simulink model "sf_slswitch_nk"  (R2020a)
settings: Solver=FixedStepAuto  StartTime=0.0  StopTime=options.T_train  FixedStep=options.dt  MaxStep=.2  RelTol=1e-3
model workspace (MAT data in the model file):
  PID_TRESH = 0.3
values from neighbouring files (symbols this model uses):
  options = trainingOptions('sgdm',      'MiniBatchSize',miniBatchSize,      'MaxEpochs',30,      'InitialLearnRate',1e-3,      'LearnRateSchedule','piecewise',      'LearnRateDropFactor',0.1,      'LearnRateDropPeriod',20,      'Shuffle','every-epoch',      'ValidationData',{XValidation,YValidation},      'ValidationFrequency',validationFrequency,      'Plots','training-progress',      'Verbose',false)    [training_lstm.m]
undefined symbols (not defined in the file or in its folder): DiscIntNeverNeededParam
libraries: neural x72, simulink x3
(part 2 of 3)

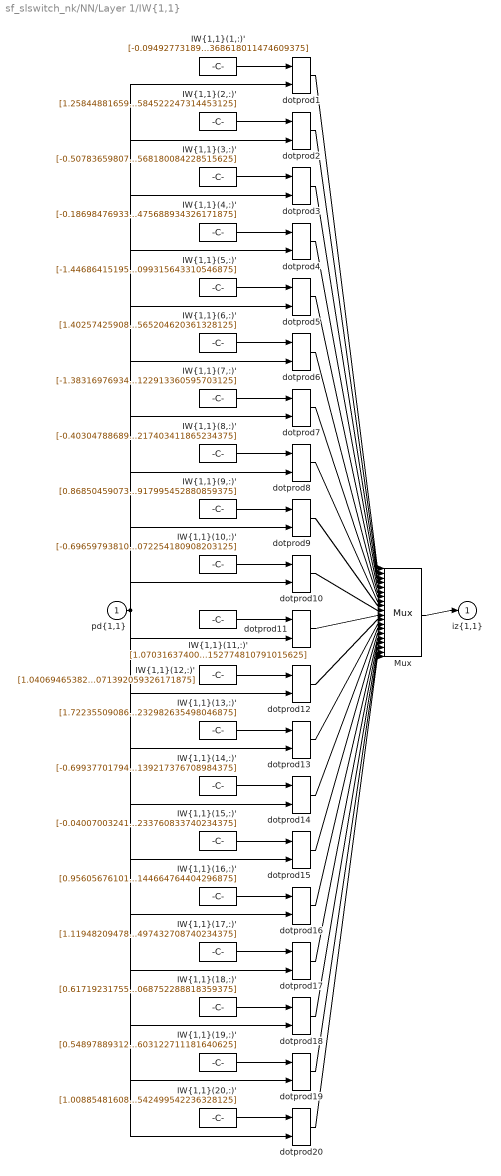
== system sf_slswitch_nk/NN/Layer 1/IW{1,1} ==
  "pd{1,1}" : Inport  PortDimensions=6
      mask Display: e = 0.06;c1 = [120 230 180]/255;c2 = ([120 230 180]+0)/(256+128);c3 = ([120 230 180]+128)/(256+128);patch([0 1 1 0],[0 0 1 1],c1);patch([0 1 1 1-e 1-e 0+e],[0 0 1 1-e 0+e 0+e],c2);patch([0 0 1 1-e 0+e 0+e],[0 1 1 1-e 1-e 0+e],c3);plot([0 1 1 0 0],[0 0 1 1 0]);
  "IW{1,1}(1,:)'" : Constant  Value=[-0.094927731895724232202837811200879514217376708984375;-1.078124816183085865617385934456251561641693115234375;-0.294993423128365128693673113957629539072513580322265625;1.256774030726915736266846579383127391338348388671875;-1.067658796670704735021217857138253748416900634765625;-0.36738733480733321012934311511344276368618011474609375]
      mask Display: e = 0.06;c1 = [120 150 230]/255;c2 = ([120 150 230]+0)/383;c3 = ([120 150 230]+128)/383;patch([0 1 1 0],[0 0 1 1],c1);patch([0 1 1 1-e 1-e 0+e],[0 0 1 1-e 0+e 0+e],c2);patch([0 0 1 1-e 0+e 0+e],[0 1 1 1-e 1-e 0+e],c3);plot([0 1 1 0 0],[0 0 1 1 0]);disp('Weights');
  "IW{1,1}(10,:)'" : Constant  Value=[-0.6965979381092519684415265146526508033275604248046875;-0.93137227491803764589661795980646274983882904052734375;-1.6314384415528950800222673933603800833225250244140625;0.32289582670247385376427473602234385907649993896484375;1.291547019617809155533905141055583953857421875;1.45726842545820733931805079919286072254180908203125]
      mask Display: e = 0.06;c1 = [120 150 230]/255;c2 = ([120 150 230]+0)/383;c3 = ([120 150 230]+128)/383;patch([0 1 1 0],[0 0 1 1],c1);patch([0 1 1 1-e 1-e 0+e],[0 0 1 1-e 0+e 0+e],c2);patch([0 0 1 1-e 0+e 0+e],[0 1 1 1-e 1-e 0+e],c3);plot([0 1 1 0 0],[0 0 1 1 0]);disp('Weights');
  "IW{1,1}(11,:)'" : Constant  Value=[1.07031637400404111559737430070526897907257080078125;-0.9847080253491229395734762874781154096126556396484375;-0.61960709489012832928978014024323783814907073974609375;1.0400372152841772521725260958191938698291778564453125;0.89700998933492004372425299152382649481296539306640625;-1.3575066104025721447357000215561129152774810791015625]
      mask Display: e = 0.06;c1 = [120 150 230]/255;c2 = ([120 150 230]+0)/383;c3 = ([120 150 230]+128)/383;patch([0 1 1 0],[0 0 1 1],c1);patch([0 1 1 1-e 1-e 0+e],[0 0 1 1-e 0+e 0+e],c2);patch([0 0 1 1-e 0+e 0+e],[0 1 1 1-e 1-e 0+e],c3);plot([0 1 1 0 0],[0 0 1 1 0]);disp('Weights');
  "IW{1,1}(12,:)'" : Constant  Value=[1.0406946538218460052149794137221761047840118408203125;-0.693594025462512586699403982493095099925994873046875;0.468858240358544176018540383665822446346282958984375;0.68547826794217259216424054102390073239803314208984375;-0.7853865691300843110411733505316078662872314453125;-1.8329776342435948333076112248818390071392059326171875]
      mask Display: e = 0.06;c1 = [120 150 230]/255;c2 = ([120 150 230]+0)/383;c3 = ([120 150 230]+128)/383;patch([0 1 1 0],[0 0 1 1],c1);patch([0 1 1 1-e 1-e 0+e],[0 0 1 1-e 0+e 0+e],c2);patch([0 0 1 1-e 0+e 0+e],[0 1 1 1-e 1-e 0+e],c3);plot([0 1 1 0 0],[0 0 1 1 0]);disp('Weights');
  "IW{1,1}(13,:)'" : Constant  Value=[1.72235509086079918716905012843199074268341064453125;-0.83361662074459186300146029680036008358001708984375;0.466763693573051419161146213809843175113201141357421875;-1.5345239974877646904616312895086593925952911376953125;-0.404560405975131487377183248099754564464092254638671875;0.421133717269054130838412675075232982635498046875]
      mask Display: e = 0.06;c1 = [120 150 230]/255;c2 = ([120 150 230]+0)/383;c3 = ([120 150 230]+128)/383;patch([0 1 1 0],[0 0 1 1],c1);patch([0 1 1 1-e 1-e 0+e],[0 0 1 1-e 0+e 0+e],c2);patch([0 0 1 1-e 0+e 0+e],[0 1 1 1-e 1-e 0+e],c3);plot([0 1 1 0 0],[0 0 1 1 0]);disp('Weights');
  "IW{1,1}(14,:)'" : Constant  Value=[-0.6993770179442133638758605229668319225311279296875;-0.67988096027652022979026469329255633056163787841796875;1.72051357171069785323425094247795641422271728515625;0.8663489352893309902725604842999018728733062744140625;0.088446533921556935720076353391050361096858978271484375;-1.4915026481155793103283713207929395139217376708984375]
      mask Display: e = 0.06;c1 = [120 150 230]/255;c2 = ([120 150 230]+0)/383;c3 = ([120 150 230]+128)/383;patch([0 1 1 0],[0 0 1 1],c1);patch([0 1 1 1-e 1-e 0+e],[0 0 1 1-e 0+e 0+e],c2);patch([0 0 1 1-e 0+e 0+e],[0 1 1 1-e 1-e 0+e],c3);plot([0 1 1 0 0],[0 0 1 1 0]);disp('Weights');
  "IW{1,1}(15,:)'" : Constant  Value=[-0.04007003241597495435399878260795958340167999267578125;-0.64990767603311094813278714354964904487133026123046875;1.57234891421088374130476950085721909999847412109375;0.9274205308829746030596652417443692684173583984375;-1.00715212796622921587186283431947231292724609375;0.50791329797469708662305265534087084233760833740234375]
      mask Display: e = 0.06;c1 = [120 150 230]/255;c2 = ([120 150 230]+0)/383;c3 = ([120 150 230]+128)/383;patch([0 1 1 0],[0 0 1 1],c1);patch([0 1 1 1-e 1-e 0+e],[0 0 1 1-e 0+e 0+e],c2);patch([0 0 1 1-e 0+e 0+e],[0 1 1 1-e 1-e 0+e],c3);plot([0 1 1 0 0],[0 0 1 1 0]);disp('Weights');
  "IW{1,1}(16,:)'" : Constant  Value=[0.9560567610105989988511510091484524309635162353515625;-0.49948812701194922336611625723890028893947601318359375;-0.353147104912922282782261618194752372801303863525390625;1.4061305339003364878180946107022464275360107421875;0.73356743970992976944245356207829900085926055908203125;0.34917156935195581279884891046094708144664764404296875]
      mask Display: e = 0.06;c1 = [120 150 230]/255;c2 = ([120 150 230]+0)/383;c3 = ([120 150 230]+128)/383;patch([0 1 1 0],[0 0 1 1],c1);patch([0 1 1 1-e 1-e 0+e],[0 0 1 1-e 0+e 0+e],c2);patch([0 0 1 1-e 0+e 0+e],[0 1 1 1-e 1-e 0+e],c3);plot([0 1 1 0 0],[0 0 1 1 0]);disp('Weights');
  "IW{1,1}(17,:)'" : Constant  Value=[1.119482094782968228940944754867814481258392333984375;-0.0866938756543667310427991878896136768162250518798828125;-0.87779953561806822737167976811178959906101226806640625;-0.11556820956189566007576985384730505757033824920654296875;-1.5384060480766901246596489727380685508251190185546875;1.2292321749120966867252491283579729497432708740234375]
      mask Display: e = 0.06;c1 = [120 150 230]/255;c2 = ([120 150 230]+0)/383;c3 = ([120 150 230]+128)/383;patch([0 1 1 0],[0 0 1 1],c1);patch([0 1 1 1-e 1-e 0+e],[0 0 1 1-e 0+e 0+e],c2);patch([0 0 1 1-e 0+e 0+e],[0 1 1 1-e 1-e 0+e],c3);plot([0 1 1 0 0],[0 0 1 1 0]);disp('Weights');
  "IW{1,1}(18,:)'" : Constant  Value=[0.61719231755529524452441592075047083199024200439453125;0.70084249385920127650706490385346114635467529296875;1.7382123869079517675118040642701089382171630859375;-0.48752271514260170359733592704287730157375335693359375;0.5146598812647040777079610052169300615787506103515625;-0.67208866071192685520685472511104308068752288818359375]
      mask Display: e = 0.06;c1 = [120 150 230]/255;c2 = ([120 150 230]+0)/383;c3 = ([120 150 230]+128)/383;patch([0 1 1 0],[0 0 1 1],c1);patch([0 1 1 1-e 1-e 0+e],[0 0 1 1-e 0+e 0+e],c2);patch([0 0 1 1-e 0+e 0+e],[0 1 1 1-e 1-e 0+e],c3);plot([0 1 1 0 0],[0 0 1 1 0]);disp('Weights');
  "IW{1,1}(19,:)'" : Constant  Value=[0.54897889312307091014275783891207538545131683349609375;0.52420835799976617241924259360530413687229156494140625;-1.331711638369591721442475318326614797115325927734375;-1.1288562296987929567393393881502561271190643310546875;0.41319496200194494317514681824832223355770111083984375;-1.146344120463029359058282352634705603122711181640625]
      mask Display: e = 0.06;c1 = [120 150 230]/255;c2 = ([120 150 230]+0)/383;c3 = ([120 150 230]+128)/383;patch([0 1 1 0],[0 0 1 1],c1);patch([0 1 1 1-e 1-e 0+e],[0 0 1 1-e 0+e 0+e],c2);patch([0 0 1 1-e 0+e 0+e],[0 1 1 1-e 1-e 0+e],c3);plot([0 1 1 0 0],[0 0 1 1 0]);disp('Weights');
  "IW{1,1}(2,:)'" : Constant  Value=[1.25844881659379570493229039129801094532012939453125;-0.45205449936551378442572968197055160999298095703125;0.23707399172482312987852992591797374188899993896484375;-0.7429016616186407961919258013949729502201080322265625;0.85319661383065203974496171213104389607906341552734375;-1.9671374360243067958009532958385534584522247314453125]
      mask Display: e = 0.06;c1 = [120 150 230]/255;c2 = ([120 150 230]+0)/383;c3 = ([120 150 230]+128)/383;patch([0 1 1 0],[0 0 1 1],c1);patch([0 1 1 1-e 1-e 0+e],[0 0 1 1-e 0+e 0+e],c2);patch([0 0 1 1-e 0+e 0+e],[0 1 1 1-e 1-e 0+e],c3);plot([0 1 1 0 0],[0 0 1 1 0]);disp('Weights');
  "IW{1,1}(20,:)'" : Constant  Value=[1.0088548160819519328157412019209004938602447509765625;-0.437510285439882851132864516330300830304622650146484375;-1.133582845050659759778000079677440226078033447265625;-0.6711148903733332726773141985177062451839447021484375;-1.06756024320649611780709165032021701335906982421875;-0.9931053506585840739973036761512048542499542236328125]
      mask Display: e = 0.06;c1 = [120 150 230]/255;c2 = ([120 150 230]+0)/383;c3 = ([120 150 230]+128)/383;patch([0 1 1 0],[0 0 1 1],c1);patch([0 1 1 1-e 1-e 0+e],[0 0 1 1-e 0+e 0+e],c2);patch([0 0 1 1-e 0+e 0+e],[0 1 1 1-e 1-e 0+e],c3);plot([0 1 1 0 0],[0 0 1 1 0]);disp('Weights');
  "IW{1,1}(3,:)'" : Constant  Value=[-0.5078365980773200671904987757443450391292572021484375;-0.98557708885253092478961889355559833347797393798828125;0.83535764937662959628283942947746254503726959228515625;-1.2674616184744886826507581645273603498935699462890625;-0.20613455194201135700637905756593681871891021728515625;1.4320485447146309443411382744670845568180084228515625]
      mask Display: e = 0.06;c1 = [120 150 230]/255;c2 = ([120 150 230]+0)/383;c3 = ([120 150 230]+128)/383;patch([0 1 1 0],[0 0 1 1],c1);patch([0 1 1 1-e 1-e 0+e],[0 0 1 1-e 0+e 0+e],c2);patch([0 0 1 1-e 0+e 0+e],[0 1 1 1-e 1-e 0+e],c3);plot([0 1 1 0 0],[0 0 1 1 0]);disp('Weights');
  "IW{1,1}(4,:)'" : Constant  Value=[-0.18698476933772523178589608505717478692531585693359375;1.5583920754114171103310582111589610576629638671875;-0.2156793839170213777922668896280811168253421783447265625;-0.72749180446784189602027481669210828840732574462890625;-1.4169092304770252166434829632635228335857391357421875;0.359325123822682612750867292561451904475688934326171875]
      mask Display: e = 0.06;c1 = [120 150 230]/255;c2 = ([120 150 230]+0)/383;c3 = ([120 150 230]+128)/383;patch([0 1 1 0],[0 0 1 1],c1);patch([0 1 1 1-e 1-e 0+e],[0 0 1 1-e 0+e 0+e],c2);patch([0 0 1 1-e 0+e 0+e],[0 1 1 1-e 1-e 0+e],c3);plot([0 1 1 0 0],[0 0 1 1 0]);disp('Weights');
  "IW{1,1}(5,:)'" : Constant  Value=[-1.4468641519511447057766417856328189373016357421875;1.0408384094097018479629923604079522192478179931640625;0.6682675190310283230843424462364055216312408447265625;-0.60434192173020873095623528570285998284816741943359375;0.278992077328215459797178255030303262174129486083984375;0.7523747497309141163412959940615110099315643310546875]
      mask Display: e = 0.06;c1 = [120 150 230]/255;c2 = ([120 150 230]+0)/383;c3 = ([120 150 230]+128)/383;patch([0 1 1 0],[0 0 1 1],c1);patch([0 1 1 1-e 1-e 0+e],[0 0 1 1-e 0+e 0+e],c2);patch([0 0 1 1-e 0+e 0+e],[0 1 1 1-e 1-e 0+e],c3);plot([0 1 1 0 0],[0 0 1 1 0]);disp('Weights');
  "IW{1,1}(6,:)'" : Constant  Value=[1.4025742590807848131362334243021905422210693359375;-0.7948216274412962523143733051256276667118072509765625;1.149026404160081948901961368392221629619598388671875;-0.2200881799925549497931598352806759066879749298095703125;-1.08693235950315969517987468861974775791168212890625;-1.2131372197811050028803947498090565204620361328125]
      mask Display: e = 0.06;c1 = [120 150 230]/255;c2 = ([120 150 230]+0)/383;c3 = ([120 150 230]+128)/383;patch([0 1 1 0],[0 0 1 1],c1);patch([0 1 1 1-e 1-e 0+e],[0 0 1 1-e 0+e 0+e],c2);patch([0 0 1 1-e 0+e 0+e],[0 1 1 1-e 1-e 0+e],c3);plot([0 1 1 0 0],[0 0 1 1 0]);disp('Weights');
  "IW{1,1}(7,:)'" : Constant  Value=[-1.3831697693493631984296143855317495763301849365234375;-0.1328306931337319696240228950046002864837646484375;0.45446086616974501470878067266312427818775177001953125;1.114971635152235851506929975585080683231353759765625;1.1100787748890772466126009021536447107791900634765625;0.367102960903916308854633143710088916122913360595703125]
      mask Display: e = 0.06;c1 = [120 150 230]/255;c2 = ([120 150 230]+0)/383;c3 = ([120 150 230]+128)/383;patch([0 1 1 0],[0 0 1 1],c1);patch([0 1 1 1-e 1-e 0+e],[0 0 1 1-e 0+e 0+e],c2);patch([0 0 1 1-e 0+e 0+e],[0 1 1 1-e 1-e 0+e],c3);plot([0 1 1 0 0],[0 0 1 1 0]);disp('Weights');
  "IW{1,1}(8,:)'" : Constant  Value=[-0.403047886898010354617127859455649740993976593017578125;0.380056563159374583005245540334726683795452117919921875;-0.99676021866128028392495252774097025394439697265625;1.296202336960913470420564408414065837860107421875;0.80139043210833371677637160246376879513263702392578125;1.1639645739591608641916309352382086217403411865234375]
      mask Display: e = 0.06;c1 = [120 150 230]/255;c2 = ([120 150 230]+0)/383;c3 = ([120 150 230]+128)/383;patch([0 1 1 0],[0 0 1 1],c1);patch([0 1 1 1-e 1-e 0+e],[0 0 1 1-e 0+e 0+e],c2);patch([0 0 1 1-e 0+e 0+e],[0 1 1 1-e 1-e 0+e],c3);plot([0 1 1 0 0],[0 0 1 1 0]);disp('Weights');
  "IW{1,1}(9,:)'" : Constant  Value=[0.86850459073675778665091229413519613444805145263671875;1.1648075479637223228479570025228895246982574462890625;0.416288169601384316909076233059749938547611236572265625;-2.027947413051115699289539406890980899333953857421875;-1.1341763634191612819535066591924987733364105224609375;1.2554216353064828748387071755132637917995452880859375]
      mask Display: e = 0.06;c1 = [120 150 230]/255;c2 = ([120 150 230]+0)/383;c3 = ([120 150 230]+128)/383;patch([0 1 1 0],[0 0 1 1],c1);patch([0 1 1 1-e 1-e 0+e],[0 0 1 1-e 0+e 0+e],c2);patch([0 0 1 1-e 0+e 0+e],[0 1 1 1-e 1-e 0+e],c3);plot([0 1 1 0 0],[0 0 1 1 0]);disp('Weights');
  Mux : Mux  Inputs=20
      mask Display: e = 0.06;c1 = [120 150 230]/255;c2 = ([120 150 230]+0)/383;c3 = ([120 150 230]+128)/383;patch([0 1 1 0],[0 0 1 1],c1);patch([0 1 1 1-e 1-e 0+e],[0 0 1 1-e 0+e 0+e],c2);patch([0 0 1 1-e 0+e 0+e],[0 1 1 1-e 1-e 0+e],c3);plot([0 1 1 0 0],[0 0 1 1 0]);disp('Mux');
  dotprod{1..20} (20 alike) : neural/Weight Functions/dotprod
  "iz{1,1}" : Outport
      mask Display: e = 0.06;c1 = [120 230 180]/255;c2 = ([120 230 180]+0)/(256+128);c3 = ([120 230 180]+128)/(256+128);patch([0 1 1 0],[0 0 1 1],c1);patch([0 1 1 1-e 1-e 0+e],[0 0 1 1-e 0+e 0+e],c2);patch([0 0 1 1-e 0+e 0+e],[0 1 1 1-e 1-e 0+e],c3);plot([0 1 1 0 0],[0 0 1 1 0]);
  wires:
  "IW{1,1}(1,:)'"/1 -> dotprod1/1
  "pd{1,1}"/1 -> dotprod1/2, dotprod2/2, dotprod3/2, dotprod4/2, dotprod5/2, dotprod6/2, dotprod7/2, dotprod8/2, dotprod9/2, dotprod10/2, dotprod11/2, dotprod12/2, dotprod13/2, dotprod14/2, dotprod15/2, dotprod16/2, dotprod17/2, dotprod18/2, dotprod19/2, dotprod20/2
  dotprod1/1 -> Mux/1
  "IW{1,1}(2,:)'"/1 -> dotprod2/1
  dotprod2/1 -> Mux/2
  "IW{1,1}(3,:)'"/1 -> dotprod3/1
  dotprod3/1 -> Mux/3
  "IW{1,1}(4,:)'"/1 -> dotprod4/1
  dotprod4/1 -> Mux/4
  "IW{1,1}(5,:)'"/1 -> dotprod5/1
  dotprod5/1 -> Mux/5
  "IW{1,1}(6,:)'"/1 -> dotprod6/1
  dotprod6/1 -> Mux/6
  "IW{1,1}(7,:)'"/1 -> dotprod7/1
  dotprod7/1 -> Mux/7
  "IW{1,1}(8,:)'"/1 -> dotprod8/1
  dotprod8/1 -> Mux/8
  "IW{1,1}(9,:)'"/1 -> dotprod9/1
  dotprod9/1 -> Mux/9
  "IW{1,1}(10,:)'"/1 -> dotprod10/1
  dotprod10/1 -> Mux/10
  "IW{1,1}(11,:)'"/1 -> dotprod11/1
  dotprod11/1 -> Mux/11
  "IW{1,1}(12,:)'"/1 -> dotprod12/1
  dotprod12/1 -> Mux/12
  "IW{1,1}(13,:)'"/1 -> dotprod13/1
  dotprod13/1 -> Mux/13
  "IW{1,1}(14,:)'"/1 -> dotprod14/1
  dotprod14/1 -> Mux/14
  "IW{1,1}(15,:)'"/1 -> dotprod15/1
  dotprod15/1 -> Mux/15
  "IW{1,1}(16,:)'"/1 -> dotprod16/1
  dotprod16/1 -> Mux/16
  "IW{1,1}(17,:)'"/1 -> dotprod17/1
  dotprod17/1 -> Mux/17
  "IW{1,1}(18,:)'"/1 -> dotprod18/1
  dotprod18/1 -> Mux/18
  "IW{1,1}(19,:)'"/1 -> dotprod19/1
  dotprod19/1 -> Mux/19
  "IW{1,1}(20,:)'"/1 -> dotprod20/1
  dotprod20/1 -> Mux/20
  Mux/1 -> "iz{1,1}"/1

== system sf_slswitch_nk/NN/Layer 2/Delays 1 ==
  "p{2}" : Inport  PortDimensions=20
      mask Display: e = 0.06;c1 = [120 230 180]/255;c2 = ([120 230 180]+0)/(256+128);c3 = ([120 230 180]+128)/(256+128);patch([0 1 1 0],[0 0 1 1],c1);patch([0 1 1 1-e 1-e 0+e],[0 0 1 1-e 0+e 0+e],c2);patch([0 0 1 1-e 0+e 0+e],[0 1 1 1-e 1-e 0+e],c3);plot([0 1 1 0 0],[0 0 1 1 0]);
  mux : Mux  Inputs=1
      mask Display: e = 0.06;c1 = [120 150 230]/255;c2 = ([120 150 230]+0)/383;c3 = ([120 150 230]+128)/383;patch([0 1 1 0],[0 0 1 1],c1);patch([0 1 1 1-e 1-e 0+e],[0 0 1 1-e 0+e 0+e],c2);patch([0 0 1 1-e 0+e 0+e],[0 1 1 1-e 1-e 0+e],c3);plot([0 1 1 0 0],[0 0 1 1 0]);disp('Mux')
  "pd{2,1}" : Outport
      mask Display: e = 0.06;c1 = [120 230 180]/255;c2 = ([120 230 180]+0)/(256+128);c3 = ([120 230 180]+128)/(256+128);patch([0 1 1 0],[0 0 1 1],c1);patch([0 1 1 1-e 1-e 0+e],[0 0 1 1-e 0+e 0+e],c2);patch([0 0 1 1-e 0+e 0+e],[0 1 1 1-e 1-e 0+e],c3);plot([0 1 1 0 0],[0 0 1 1 0]);
  wires:
  "p{2}"/1 -> mux/1
  mux/1 -> "pd{2,1}"/1

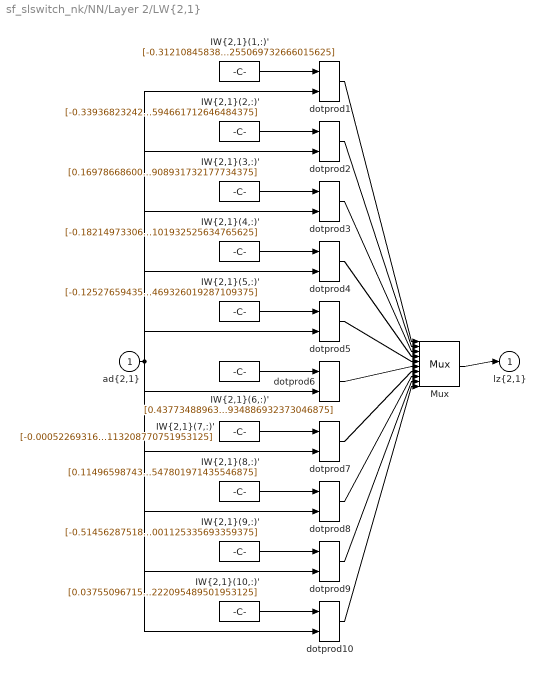
== system sf_slswitch_nk/NN/Layer 2/LW{2,1} ==
  "ad{2,1}" : Inport  PortDimensions=20
      mask Display: e = 0.06;c1 = [120 230 180]/255;c2 = ([120 230 180]+0)/(256+128);c3 = ([120 230 180]+128)/(256+128);patch([0 1 1 0],[0 0 1 1],c1);patch([0 1 1 1-e 1-e 0+e],[0 0 1 1-e 0+e 0+e],c2);patch([0 0 1 1-e 0+e 0+e],[0 1 1 1-e 1-e 0+e],c3);plot([0 1 1 0 0],[0 0 1 1 0]);
  "IW{2,1}(1,:)'" : Constant  Value=[-0.312108458380050468594646417841431684792041778564453125;0.5441555455421831499762674866360612213611602783203125;0.51222797301980194095705201107193715870380401611328125;-0.274007683295291737390897424120339564979076385498046875;-0.27163138401487374462561774635105393826961517333984375;0.96630982262287423711910605561570264399051666259765625;-0.2143163089321049319391221388286794535815715789794921875;0.288545705457057988230218370517832227051258087158203125;-1.576748069000661001126672999816946685314178466796875;-0.270422245520684001451883204936166293919086456298828125;-0.433935019236317998103658055697451345622539520263671875;-0.574312829446991468529404301079921424388885498046875;0.370195654695306630710405215722857974469661712646484375;-0.251239629887962834242642884419183246791362762451171875;0.37455523898456399845002806614502333104610443115234375;0.010231119911725379545419656324156676419079303741455078125;-0.29258149348964501701431117908214218914508819580078125;0.83514303689856161927451694282353855669498443603515625;0.159824137382432673870624739720369689166545867919921875;-0.09865937932771874641080245282864780165255069732666015625]
      mask Display: e = 0.06;c1 = [120 150 230]/255;c2 = ([120 150 230]+0)/383;c3 = ([120 150 230]+128)/383;patch([0 1 1 0],[0 0 1 1],c1);patch([0 1 1 1-e 1-e 0+e],[0 0 1 1-e 0+e 0+e],c2);patch([0 0 1 1-e 0+e 0+e],[0 1 1 1-e 1-e 0+e],c3);plot([0 1 1 0 0],[0 0 1 1 0]);disp('weights');
  "IW{2,1}(10,:)'" : Constant  Value=[0.037550967153765983652657922675643931142985820770263671875;-0.39674968881058825243002274874015711247920989990234375;-0.368650493002415757803902351952274329960346221923828125;0.339420061314512244710073218811885453760623931884765625;0.04272952323082035430701353106996975839138031005859375;0.1677611241168373290566506739196483977138996124267578125;-0.581904200521492054321015530149452388286590576171875;-0.437018345504167127213435151134035550057888031005859375;-0.63107799727578406390193777042441070079803466796875;0.1195605054390375954209702058506081812083721160888671875;-0.446277103641889050233970692715956829488277435302734375;-0.2366272690103541076478421700812759809195995330810546875;0.6794572985363969142014184399158693850040435791015625;-0.2020210178180097126965364395800861530005931854248046875;-0.419464342985588933832019620240316726267337799072265625;-0.3818445042545242085196832704241387546062469482421875;0.44299207277223418000033916541724465787410736083984375;0.1404220888878456030557373424016986973583698272705078125;-0.347946882755673925213812935908208601176738739013671875;-0.69824101307660246806818804543581791222095489501953125]
      mask Display: e = 0.06;c1 = [120 150 230]/255;c2 = ([120 150 230]+0)/383;c3 = ([120 150 230]+128)/383;patch([0 1 1 0],[0 0 1 1],c1);patch([0 1 1 1-e 1-e 0+e],[0 0 1 1-e 0+e 0+e],c2);patch([0 0 1 1-e 0+e 0+e],[0 1 1 1-e 1-e 0+e],c3);plot([0 1 1 0 0],[0 0 1 1 0]);disp('weights');
  "IW{2,1}(2,:)'" : Constant  Value=[-0.33936823242451541471353948509204201400279998779296875;-0.34848047594259601300592521511134691536426544189453125;0.07410024833324206638973663530123303644359111785888671875;-0.33730624040655710071945350136957131326198577880859375;-0.2529673365591549316633290800382383167743682861328125;0.2062167147281236678768578940434963442385196685791015625;-0.041988422915805345692064065588056109845638275146484375;-0.41618110065184443779884304603911004960536956787109375;-0.56851599639557537368972361946362070739269256591796875;0.229120695052757394893916398359579034149646759033203125;-0.97561161741273438874344492433010600507259368896484375;-0.440193747154081826966631751929526217281818389892578125;0.310745364357229159057993683745735324919223785400390625;0.61191010488567643132995499399839900434017181396484375;0.52355695033273319527467037914902903139591217041015625;0.425691824582956013234280590040725655853748321533203125;0.254920810689424015560433645077864639461040496826171875;-0.1603571414800424310698190311086364090442657470703125;-0.173730812973854009673146947534405626356601715087890625;0.319182632807168020772081717950641177594661712646484375]
      mask Display: e = 0.06;c1 = [120 150 230]/255;c2 = ([120 150 230]+0)/383;c3 = ([120 150 230]+128)/383;patch([0 1 1 0],[0 0 1 1],c1);patch([0 1 1 1-e 1-e 0+e],[0 0 1 1-e 0+e 0+e],c2);patch([0 0 1 1-e 0+e 0+e],[0 1 1 1-e 1-e 0+e],c3);plot([0 1 1 0 0],[0 0 1 1 0]);disp('weights');
  "IW{2,1}(3,:)'" : Constant  Value=[0.169786686003889852880632815868011675775051116943359375;0.415886541774417584083067822575685568153858184814453125;-0.330538305032426593665917380349128507077693939208984375;-0.028626283154292379851124650258498149923980236053466796875;0.30402558769584298037358394140028394758701324462890625;-0.857771501207724273996291231014765799045562744140625;-0.3890543598058984198218013261794112622737884521484375;-0.100276383676814351275652370532043278217315673828125;-0.290737013511904507367944461293518543243408203125;-0.476043951880538107612750309272087179124355316162109375;-0.9842286834534645922900608638883568346500396728515625;-0.456667796184613561383258684145403094589710235595703125;0.1513208706193082953017636782533372752368450164794921875;-0.53339199606164466871405238634906709194183349609375;-0.2452044981374068288726419950762647204101085662841796875;-0.9063632216929813356642853250377811491489410400390625;0.06635392764725907277512106929862056858837604522705078125;0.65611261000505682883243707692599855363368988037109375;0.13324597163405249578005395960644818842411041259765625;0.36409709231659093120470060966908931732177734375]
      mask Display: e = 0.06;c1 = [120 150 230]/255;c2 = ([120 150 230]+0)/383;c3 = ([120 150 230]+128)/383;patch([0 1 1 0],[0 0 1 1],c1);patch([0 1 1 1-e 1-e 0+e],[0 0 1 1-e 0+e 0+e],c2);patch([0 0 1 1-e 0+e 0+e],[0 1 1 1-e 1-e 0+e],c3);plot([0 1 1 0 0],[0 0 1 1 0]);disp('weights');
  "IW{2,1}(4,:)'" : Constant  Value=[-0.18214973306806869768337264758883975446224212646484375;-0.017452343753403619375230704235946177504956722259521484375;-0.8870982173297987660731678261072374880313873291015625;0.16288622005385844371261327978572808206081390380859375;-0.537107721134259197270921504241414368152618408203125;0.150301090648870483423849009341211058199405670166015625;0.1278022231531671659698901066803955473005771636962890625;0.54439484641013680121801598943420685827732086181640625;-0.5539834596486856721497815669863484799861907958984375;-1.0069720719420283128187065813108347356319427490234375;0.0848256172996120216822646398213692009449005126953125;-0.02750637080596367300966420543772983364760875701904296875;0.78511679030030301351672505916212685406208038330078125;0.231720832869142967513909070476074703037738800048828125;-0.62521938437448876246804729817085899412631988525390625;-0.145224909523523126875232946986216120421886444091796875;0.4013106154437888761776775936596095561981201171875;0.06603150518927795864509988632562453858554363250732421875;0.2205714314447675683528160561763797886669635772705078125;-0.1807387550152802779823701939676539041101932525634765625]
      mask Display: e = 0.06;c1 = [120 150 230]/255;c2 = ([120 150 230]+0)/383;c3 = ([120 150 230]+128)/383;patch([0 1 1 0],[0 0 1 1],c1);patch([0 1 1 1-e 1-e 0+e],[0 0 1 1-e 0+e 0+e],c2);patch([0 0 1 1-e 0+e 0+e],[0 1 1 1-e 1-e 0+e],c3);plot([0 1 1 0 0],[0 0 1 1 0]);disp('weights');
  "IW{2,1}(5,:)'" : Constant  Value=[-0.12527659435284987932135436494718305766582489013671875;0.388803336360501849977566735105938278138637542724609375;-0.223245802381738800423960356056340970098972320556640625;0.1607999992858925308869544323897571302950382232666015625;0.36306437130872926122293620210257358849048614501953125;-0.020684689599425397366072587601593113504350185394287109375;-0.407071273978032499574197800029651261866092681884765625;0.4916948061555876936523645781562663614749908447265625;0.25004038023133567936184817881439812481403350830078125;0.844105909005153254298647880204953253269195556640625;-0.160798229308410756122071916252025403082370758056640625;0.81747019297968226414496939469245262444019317626953125;0.266518468814056663784839429354178719222545623779296875;0.11132057729270317114611543729552067816257476806640625;-0.321379858291721109964100833167321979999542236328125;0.49882024757255971625369284083717502653598785400390625;0.320636234721343893472322861271095462143421173095703125;0.54948076042705140675792563342838548123836517333984375;-0.2207993587464956719568220933069824241101741790771484375;-0.0388368831956470150768012672415352426469326019287109375]
      mask Display: e = 0.06;c1 = [120 150 230]/255;c2 = ([120 150 230]+0)/383;c3 = ([120 150 230]+128)/383;patch([0 1 1 0],[0 0 1 1],c1);patch([0 1 1 1-e 1-e 0+e],[0 0 1 1-e 0+e 0+e],c2);patch([0 0 1 1-e 0+e 0+e],[0 1 1 1-e 1-e 0+e],c3);plot([0 1 1 0 0],[0 0 1 1 0]);disp('weights');
  "IW{2,1}(6,:)'" : Constant  Value=[0.437734889632903134693009405964403413236141204833984375;0.81505779354598895114492052016430534422397613525390625;-0.161380038785271739953941505518741905689239501953125;0.08275408714318742420257279945872141979634761810302734375;-0.042217756226518188267249342970899306237697601318359375;-0.332830965470693296293092089399578981101512908935546875;0.37144879719026990816388433813699521124362945556640625;-0.60499859732638316955899426830001175403594970703125;0.0986885039169800304392765610828064382076263427734375;0.169509414044340889216044843124109320342540740966796875;0.6666425895478536034488570294342935085296630859375;0.374151528121305199103829863815917633473873138427734375;-0.038415197720902127809239345879177562892436981201171875;0.70771130339965837574567331103025935590267181396484375;0.08303721002319182364903582538318005390465259552001953125;-0.6360384718541027826432809888501651585102081298828125;0.113950829401357534020888806480797939002513885498046875;-0.30404868245821681238538758407230488955974578857421875;0.66912830743871543059952955445623956620693206787109375;-0.0627540806988797494891940687011810950934886932373046875]
      mask Display: e = 0.06;c1 = [120 150 230]/255;c2 = ([120 150 230]+0)/383;c3 = ([120 150 230]+128)/383;patch([0 1 1 0],[0 0 1 1],c1);patch([0 1 1 1-e 1-e 0+e],[0 0 1 1-e 0+e 0+e],c2);patch([0 0 1 1-e 0+e 0+e],[0 1 1 1-e 1-e 0+e],c3);plot([0 1 1 0 0],[0 0 1 1 0]);disp('weights');
  "IW{2,1}(7,:)'" : Constant  Value=[-0.000522693160811628192152777927503848331980407238006591796875;-0.417303480428247552946885434721480123698711395263671875;0.0272020120865798416265324277674153563566505908966064453125;0.11002153263502745250690395550918765366077423095703125;0.5362334457145740973516012672916986048221588134765625;-0.228217982403624730647351270818035118281841278076171875;-0.29896993646603042815712569790775887668132781982421875;-0.00952933825981709670127628442060085944831371307373046875;-0.2391413120484424670308953864150680601596832275390625;-0.24072353443058336353033155319280922412872314453125;0.179732425298842368732721297419629991054534912109375;0.64016825481440253753362412680871784687042236328125;0.2265880994467727449492855384960421361029148101806640625;0.71421967935661123672019812147482298314571380615234375;0.86527188415422084943884328822605311870574951171875;0.71404019800633677927947928765206597745418548583984375;-0.58292914869512768571979677290073595941066741943359375;0.37044566859840954986538008597563020884990692138671875;-0.02585738246435197174033504552426165901124477386474609375;0.226493798301785009829956152316299267113208770751953125]
      mask Display: e = 0.06;c1 = [120 150 230]/255;c2 = ([120 150 230]+0)/383;c3 = ([120 150 230]+128)/383;patch([0 1 1 0],[0 0 1 1],c1);patch([0 1 1 1-e 1-e 0+e],[0 0 1 1-e 0+e 0+e],c2);patch([0 0 1 1-e 0+e 0+e],[0 1 1 1-e 1-e 0+e],c3);plot([0 1 1 0 0],[0 0 1 1 0]);disp('weights');
  "IW{2,1}(8,:)'" : Constant  Value=[0.11496598743822299126815522640754352323710918426513671875;0.383639646601758144139893147439579479396343231201171875;0.0082420861548074368652105903265692177228629589080810546875;-0.387428183655450009137410916082444600760936737060546875;0.303171278931018528535190625916584394872188568115234375;0.2128858578256208888834777326337643899023532867431640625;0.6154450129666628743763112652231939136981964111328125;0.1465994795495134395135750082772574387490749359130859375;0.6130245510118685903222512934007681906223297119140625;0.49857614772025871108240835383185185492038726806640625;-0.73779954593630225900824370910413563251495361328125;-0.2973771482797697984779006219469010829925537109375;-0.61163433675855538584897885812097229063510894775390625;-0.62313218853402163599497498580603860318660736083984375;-0.2922311663186218932963811312220059335231781005859375;-0.2191077804158062247719129800316295586526393890380859375;0.50707870916798147842285970909870229661464691162109375;0.533914118569158713256683768122456967830657958984375;0.5050295162271822846378199756145477294921875;-0.403012247309771254322185995988547801971435546875]
      mask Display: e = 0.06;c1 = [120 150 230]/255;c2 = ([120 150 230]+0)/383;c3 = ([120 150 230]+128)/383;patch([0 1 1 0],[0 0 1 1],c1);patch([0 1 1 1-e 1-e 0+e],[0 0 1 1-e 0+e 0+e],c2);patch([0 0 1 1-e 0+e 0+e],[0 1 1 1-e 1-e 0+e],c3);plot([0 1 1 0 0],[0 0 1 1 0]);disp('weights');
  "IW{2,1}(9,:)'" : Constant  Value=[-0.51456287518051235796434639269136823713779449462890625;0.01245736790822498697706155468267752439714968204498291015625;-0.310614614470953231961658502768841572105884552001953125;-0.50433972192240250631556364169227890670299530029296875;0.25662975887280647935284605409833602607250213623046875;0.1836399798032303520844976674197823740541934967041015625;0.214280818823563590225234065655968151986598968505859375;-0.416958092706061933530037322270800359547138214111328125;0.1821845094510890217254228673482430167496204376220703125;0.362020344534043747586338213295675814151763916015625;0.042838067963877519972459850805535097606480121612548828125;0.524739879167395173453769530169665813446044921875;-0.44358762172595278538977936477749608457088470458984375;-0.285579690590211765499617513341945596039295196533203125;0.2743440981415850021818414461449719965457916259765625;0.0591808388211370328679805652427603490650653839111328125;-0.35963744736276670455055182173964567482471466064453125;-0.458928160499127935079144435803755186498165130615234375;0.07836054962490184017109839942349935881793498992919921875;-0.5099601369221742341864000991336070001125335693359375]
      mask Display: e = 0.06;c1 = [120 150 230]/255;c2 = ([120 150 230]+0)/383;c3 = ([120 150 230]+128)/383;patch([0 1 1 0],[0 0 1 1],c1);patch([0 1 1 1-e 1-e 0+e],[0 0 1 1-e 0+e 0+e],c2);patch([0 0 1 1-e 0+e 0+e],[0 1 1 1-e 1-e 0+e],c3);plot([0 1 1 0 0],[0 0 1 1 0]);disp('weights');
  Mux : Mux  Inputs=10
      mask Display: e = 0.06;c1 = [120 150 230]/255;c2 = ([120 150 230]+0)/383;c3 = ([120 150 230]+128)/383;patch([0 1 1 0],[0 0 1 1],c1);patch([0 1 1 1-e 1-e 0+e],[0 0 1 1-e 0+e 0+e],c2);patch([0 0 1 1-e 0+e 0+e],[0 1 1 1-e 1-e 0+e],c3);plot([0 1 1 0 0],[0 0 1 1 0]);disp('Mux');
  dotprod{1..10} (10 alike) : neural/Weight Functions/dotprod
  "lz{2,1}" : Outport
      mask Display: e = 0.06;c1 = [120 230 180]/255;c2 = ([120 230 180]+0)/(256+128);c3 = ([120 230 180]+128)/(256+128);patch([0 1 1 0],[0 0 1 1],c1);patch([0 1 1 1-e 1-e 0+e],[0 0 1 1-e 0+e 0+e],c2);patch([0 0 1 1-e 0+e 0+e],[0 1 1 1-e 1-e 0+e],c3);plot([0 1 1 0 0],[0 0 1 1 0]);
  wires:
  "IW{2,1}(1,:)'"/1 -> dotprod1/1
  "ad{2,1}"/1 -> dotprod1/2, dotprod2/2, dotprod3/2, dotprod4/2, dotprod5/2, dotprod6/2, dotprod7/2, dotprod8/2, dotprod9/2, dotprod10/2
  dotprod1/1 -> Mux/1
  "IW{2,1}(2,:)'"/1 -> dotprod2/1
  dotprod2/1 -> Mux/2
  "IW{2,1}(3,:)'"/1 -> dotprod3/1
  dotprod3/1 -> Mux/3
  "IW{2,1}(4,:)'"/1 -> dotprod4/1
  dotprod4/1 -> Mux/4
  "IW{2,1}(5,:)'"/1 -> dotprod5/1
  dotprod5/1 -> Mux/5
  "IW{2,1}(6,:)'"/1 -> dotprod6/1
  dotprod6/1 -> Mux/6
  "IW{2,1}(7,:)'"/1 -> dotprod7/1
  dotprod7/1 -> Mux/7
  "IW{2,1}(8,:)'"/1 -> dotprod8/1
  dotprod8/1 -> Mux/8
  "IW{2,1}(9,:)'"/1 -> dotprod9/1
  dotprod9/1 -> Mux/9
  "IW{2,1}(10,:)'"/1 -> dotprod10/1
  dotprod10/1 -> Mux/10
  Mux/1 -> "lz{2,1}"/1

== system sf_slswitch_nk/NN/Layer 3/Delays 1 ==
  "p{3}" : Inport  PortDimensions=10
      mask Display: e = 0.06;c1 = [120 230 180]/255;c2 = ([120 230 180]+0)/(256+128);c3 = ([120 230 180]+128)/(256+128);patch([0 1 1 0],[0 0 1 1],c1);patch([0 1 1 1-e 1-e 0+e],[0 0 1 1-e 0+e 0+e],c2);patch([0 0 1 1-e 0+e 0+e],[0 1 1 1-e 1-e 0+e],c3);plot([0 1 1 0 0],[0 0 1 1 0]);
  mux : Mux  Inputs=1
      mask Display: e = 0.06;c1 = [120 150 230]/255;c2 = ([120 150 230]+0)/383;c3 = ([120 150 230]+128)/383;patch([0 1 1 0],[0 0 1 1],c1);patch([0 1 1 1-e 1-e 0+e],[0 0 1 1-e 0+e 0+e],c2);patch([0 0 1 1-e 0+e 0+e],[0 1 1 1-e 1-e 0+e],c3);plot([0 1 1 0 0],[0 0 1 1 0]);disp('Mux')
  "pd{3,2}" : Outport
      mask Display: e = 0.06;c1 = [120 230 180]/255;c2 = ([120 230 180]+0)/(256+128);c3 = ([120 230 180]+128)/(256+128);patch([0 1 1 0],[0 0 1 1],c1);patch([0 1 1 1-e 1-e 0+e],[0 0 1 1-e 0+e 0+e],c2);patch([0 0 1 1-e 0+e 0+e],[0 1 1 1-e 1-e 0+e],c3);plot([0 1 1 0 0],[0 0 1 1 0]);
  wires:
  "p{3}"/1 -> mux/1
  mux/1 -> "pd{3,2}"/1

== system sf_slswitch_nk/NN/Layer 3/LW{3,2} ==
  "ad{3,2}" : Inport  PortDimensions=10
      mask Display: e = 0.06;c1 = [120 230 180]/255;c2 = ([120 230 180]+0)/(256+128);c3 = ([120 230 180]+128)/(256+128);patch([0 1 1 0],[0 0 1 1],c1);patch([0 1 1 1-e 1-e 0+e],[0 0 1 1-e 0+e 0+e],c2);patch([0 0 1 1-e 0+e 0+e],[0 1 1 1-e 1-e 0+e],c3);plot([0 1 1 0 0],[0 0 1 1 0]);
  "IW{3,2}(1,:)'" : Constant  Value=[-1.377048614898999545630431384779512882232666015625;0.91311695346060606226501477067358791828155517578125;-0.922992159589669736163841662346385419368743896484375;0.97291101707597704706387276019086129963397979736328125;1.189735678010896524625650272355414927005767822265625;1.038806680752831113068168633617460727691650390625;1.00512909747626366652184515260159969329833984375;1.113651008914276818728694706805981695652008056640625;-0.351258267448357919260359949475969187915325164794921875;-0.474044713743236034719785720881191082298755645751953125]
      mask Display: e = 0.06;c1 = [120 150 230]/255;c2 = ([120 150 230]+0)/383;c3 = ([120 150 230]+128)/383;patch([0 1 1 0],[0 0 1 1],c1);patch([0 1 1 1-e 1-e 0+e],[0 0 1 1-e 0+e 0+e],c2);patch([0 0 1 1-e 0+e 0+e],[0 1 1 1-e 1-e 0+e],c3);plot([0 1 1 0 0],[0 0 1 1 0]);disp('weights');
  Mux : Mux  Inputs=1
      mask Display: e = 0.06;c1 = [120 150 230]/255;c2 = ([120 150 230]+0)/383;c3 = ([120 150 230]+128)/383;patch([0 1 1 0],[0 0 1 1],c1);patch([0 1 1 1-e 1-e 0+e],[0 0 1 1-e 0+e 0+e],c2);patch([0 0 1 1-e 0+e 0+e],[0 1 1 1-e 1-e 0+e],c3);plot([0 1 1 0 0],[0 0 1 1 0]);disp('Mux');
  dotprod1 : neural/Weight Functions/dotprod
  "lz{3,2}" : Outport
      mask Display: e = 0.06;c1 = [120 230 180]/255;c2 = ([120 230 180]+0)/(256+128);c3 = ([120 230 180]+128)/(256+128);patch([0 1 1 0],[0 0 1 1],c1);patch([0 1 1 1-e 1-e 0+e],[0 0 1 1-e 0+e 0+e],c2);patch([0 0 1 1-e 0+e 0+e],[0 1 1 1-e 1-e 0+e],c3);plot([0 1 1 0 0],[0 0 1 1 0]);
  wires:
  "IW{3,2}(1,:)'"/1 -> dotprod1/1
  "ad{3,2}"/1 -> dotprod1/2
  dotprod1/1 -> Mux/1
  Mux/1 -> "lz{3,2}"/1

== system sf_slswitch_nk/NN_cex_1/Layer 1/Delays 1 ==
  "p{1}" : Inport  PortDimensions=6
      mask Display: e = 0.06;c1 = [120 230 180]/255;c2 = ([120 230 180]+0)/(256+128);c3 = ([120 230 180]+128)/(256+128);patch([0 1 1 0],[0 0 1 1],c1);patch([0 1 1 1-e 1-e 0+e],[0 0 1 1-e 0+e 0+e],c2);patch([0 0 1 1-e 0+e 0+e],[0 1 1 1-e 1-e 0+e],c3);plot([0 1 1 0 0],[0 0 1 1 0]);
  mux : Mux  Inputs=1
      mask Display: e = 0.06;c1 = [120 150 230]/255;c2 = ([120 150 230]+0)/383;c3 = ([120 150 230]+128)/383;patch([0 1 1 0],[0 0 1 1],c1);patch([0 1 1 1-e 1-e 0+e],[0 0 1 1-e 0+e 0+e],c2);patch([0 0 1 1-e 0+e 0+e],[0 1 1 1-e 1-e 0+e],c3);plot([0 1 1 0 0],[0 0 1 1 0]);disp('Mux')
  "pd{1,1}" : Outport
      mask Display: e = 0.06;c1 = [120 230 180]/255;c2 = ([120 230 180]+0)/(256+128);c3 = ([120 230 180]+128)/(256+128);patch([0 1 1 0],[0 0 1 1],c1);patch([0 1 1 1-e 1-e 0+e],[0 0 1 1-e 0+e 0+e],c2);patch([0 0 1 1-e 0+e 0+e],[0 1 1 1-e 1-e 0+e],c3);plot([0 1 1 0 0],[0 0 1 1 0]);
  wires:
  "p{1}"/1 -> mux/1
  mux/1 -> "pd{1,1}"/1
